simulink model "DiagnosPipeline"  (R2023b)
settings: Solver=VariableStepAuto  StartTime=0.0  StopTime=10.0  RelTol=1e-3
model workspace (MAT data in the model file):
  Signal = Simulink.ValueType
  Signal.Unit = 'V'
settings Model: Creator=user  LastModifiedBy=user

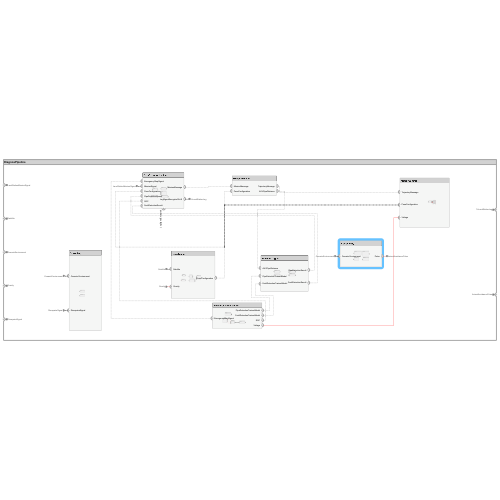
[thumbnail: Simulink's stored preview of the top-level diagram]
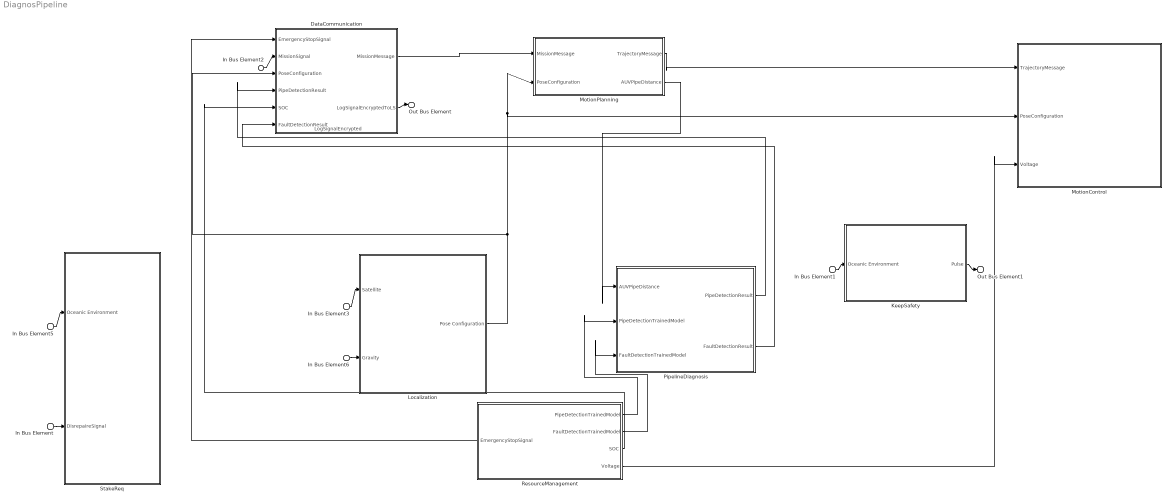
== system DiagnosPipeline ==
  In Bus Element2 : Inport  PortName=LandStationMissionSignal
  In Bus Element3 : Inport  Port=2  PortName=Satellite
  In Bus Element1 : Inport  Port=3  PortName=OceanicEnvironment
  In Bus Element5 : Inport  Port=3  PortName=OceanicEnvironment
  In Bus Element6 : Inport  Port=4  PortName=Gravity
  In Bus Element : Inport  Port=5  PortName=DisrepaireSignal
  DataCommunication : Subsystem
      settings: PortSchema="{\"entries\":[{\"content\":{\"headerSize\":26,\"margin\":15,\"minimumSpacing\":25,\"sides\":[{\"content\":{\"connectorIds\":[\"In7\",\"In2\",\"In3\",\"In4\",\"In5\",\"In6\"]},\"type\":\"ConnectorPlacement.EquallySpacedRectSide\",\"uuid\":\"b3d58345-43be-4317-860a-c8f4bed21ded\"},{\"content\":{\"connectorIds\":[\"Out1\",\"Out2\"],\"side\":\"RIGHT\"},\"type\":\"ConnectorPlacement.EquallySpacedRectSide\",\"uuid\":\"08e8d4ff-ef02-4699-9445-63f561e5af0c\"},{\"content\":{\"side\":\"TOP\"},\"type\":\"ConnectorPlacement.EquallySpacedRectSide\",\"uuid\":\"7d1ef7df-3e88-4641-86fc-bf7d4b5fe69f\"},{\"content\":{\"connectorIds\":[\"In1\"],\"side\":\"BOTTOM\"},\"type\":\"ConnectorPlacement.EquallySpacedRectSide\",\"uuid\":\"bd1e44a0-91aa-4375-ad49-10f8b22e6d3f\"}]},\"type\":\"ConnectorPlacement.EquallySpacedConnector\",\"uuid\":\"d738e7d3-0b43-4bd6-b335-43d88195508e\"}],\"packageUris\":[\"http://schema.mathworks.com/mf0/Connector/R2020b\"],\"version\":\"1.0\"}"
  KeepSafety : Subsystem
      settings: PortSchema="{\"entries\":[{\"content\":{\"headerSize\":26,\"margin\":15,\"minimumSpacing\":25,\"sides\":[{\"content\":{\"connectorIds\":[\"In1\"]},\"type\":\"ConnectorPlacement.EquallySpacedRectSide\",\"uuid\":\"b3d58345-43be-4317-860a-c8f4bed21ded\"},{\"content\":{\"connectorIds\":[\"Out1\"],\"side\":\"RIGHT\"},\"type\":\"ConnectorPlacement.EquallySpacedRectSide\",\"uuid\":\"08e8d4ff-ef02-4699-9445-63f561e5af0c\"},{\"content\":{\"side\":\"TOP\"},\"type\":\"ConnectorPlacement.EquallySpacedRectSide\",\"uuid\":\"7d1ef7df-3e88-4641-86fc-bf7d4b5fe69f\"}]},\"type\":\"ConnectorPlacement.EquallySpacedConnector\",\"uuid\":\"d738e7d3-0b43-4bd6-b335-43d88195508e\"}],\"packageUris\":[\"http://schema.mathworks.com/mf0/Connector/R2020b\"],\"version\":\"1.0\"}"
  Localization : Subsystem
      settings: PortSchema="{\"entries\":[{\"content\":{\"headerSize\":26,\"margin\":15,\"minimumSpacing\":25,\"sides\":[{\"content\":{\"connectorIds\":[\"In1\",\"In2\"]},\"type\":\"ConnectorPlacement.EquallySpacedRectSide\",\"uuid\":\"b3d58345-43be-4317-860a-c8f4bed21ded\"},{\"content\":{\"connectorIds\":[\"Out1\"],\"side\":\"RIGHT\"},\"type\":\"ConnectorPlacement.EquallySpacedRectSide\",\"uuid\":\"08e8d4ff-ef02-4699-9445-63f561e5af0c\"},{\"content\":{\"side\":\"TOP\"},\"type\":\"ConnectorPlacement.EquallySpacedRectSide\",\"uuid\":\"7d1ef7df-3e88-4641-86fc-bf7d4b5fe69f\"}]},\"type\":\"ConnectorPlacement.EquallySpacedConnector\",\"uuid\":\"d738e7d3-0b43-4bd6-b335-43d88195508e\"}],\"packageUris\":[\"http://schema.mathworks.com/mf0/Connector/R2020b\"],\"version\":\"1.0\"}"
  MotionControl : Subsystem
      settings: PortSchema="{\"entries\":[{\"content\":{\"headerSize\":26,\"margin\":15,\"minimumSpacing\":25,\"sides\":[{\"content\":{\"connectorIds\":[\"In1\",\"In2\",\"In3\"]},\"type\":\"ConnectorPlacement.EquallySpacedRectSide\",\"uuid\":\"2febbb42-d1b9-4a88-a98c-82119c43dfae\"},{\"content\":{\"side\":\"RIGHT\"},\"type\":\"ConnectorPlacement.EquallySpacedRectSide\",\"uuid\":\"6c566bdb-e273-46e8-952f-8993688d3046\"},{\"content\":{\"side\":\"TOP\"},\"type\":\"ConnectorPlacement.EquallySpacedRectSide\",\"uuid\":\"e45a7293-b6d9-4b29-b5bd-510d1f0460b1\"}]},\"type\":\"ConnectorPlacement.EquallySpacedConnector\",\"uuid\":\"1be34787-3cbc-414b-91e0-fdbde8ab0ed9\"}],\"packageUris\":[\"http://schema.mathworks.com/mf0/Connector/R2020b\"],\"version\":\"1.0\"}"
  MotionPlanning : Subsystem
      settings: PortSchema="{\"entries\":[{\"content\":{\"headerSize\":26,\"margin\":15,\"minimumSpacing\":25,\"sides\":[{\"content\":{\"connectorIds\":[\"In1\",\"In2\"]},\"type\":\"ConnectorPlacement.EquallySpacedRectSide\",\"uuid\":\"b3d58345-43be-4317-860a-c8f4bed21ded\"},{\"content\":{\"connectorIds\":[\"Out1\",\"Out2\"],\"side\":\"RIGHT\"},\"type\":\"ConnectorPlacement.EquallySpacedRectSide\",\"uuid\":\"08e8d4ff-ef02-4699-9445-63f561e5af0c\"},{\"content\":{\"side\":\"TOP\"},\"type\":\"ConnectorPlacement.EquallySpacedRectSide\",\"uuid\":\"7d1ef7df-3e88-4641-86fc-bf7d4b5fe69f\"}]},\"type\":\"ConnectorPlacement.EquallySpacedConnector\",\"uuid\":\"d738e7d3-0b43-4bd6-b335-43d88195508e\"}],\"packageUris\":[\"http://schema.mathworks.com/mf0/Connector/R2020b\"],\"version\":\"1.0\"}"
  PipelineDiagnosis : Subsystem
      settings: PortSchema="{\"entries\":[{\"content\":{\"headerSize\":26,\"margin\":15,\"minimumSpacing\":25,\"sides\":[{\"content\":{\"connectorIds\":[\"In1\",\"In2\",\"In3\"]},\"type\":\"ConnectorPlacement.EquallySpacedRectSide\",\"uuid\":\"b3d58345-43be-4317-860a-c8f4bed21ded\"},{\"content\":{\"connectorIds\":[\"Out1\",\"Out2\"],\"side\":\"RIGHT\"},\"type\":\"ConnectorPlacement.EquallySpacedRectSide\",\"uuid\":\"08e8d4ff-ef02-4699-9445-63f561e5af0c\"},{\"content\":{\"side\":\"TOP\"},\"type\":\"ConnectorPlacement.EquallySpacedRectSide\",\"uuid\":\"7d1ef7df-3e88-4641-86fc-bf7d4b5fe69f\"}]},\"type\":\"ConnectorPlacement.EquallySpacedConnector\",\"uuid\":\"d738e7d3-0b43-4bd6-b335-43d88195508e\"}],\"packageUris\":[\"http://schema.mathworks.com/mf0/Connector/R2020b\"],\"version\":\"1.0\"}"
  ResourceManagement : Subsystem
      settings: PortSchema="{\"entries\":[{\"content\":{\"headerSize\":26,\"margin\":15,\"minimumSpacing\":25,\"sides\":[{\"content\":{\"connectorIds\":[\"Out5\"]},\"type\":\"ConnectorPlacement.EquallySpacedRectSide\",\"uuid\":\"b3d58345-43be-4317-860a-c8f4bed21ded\"},{\"content\":{\"connectorIds\":[\"Out1\",\"Out2\",\"Out3\",\"Out4\"],\"side\":\"RIGHT\"},\"type\":\"ConnectorPlacement.EquallySpacedRectSide\",\"uuid\":\"08e8d4ff-ef02-4699-9445-63f561e5af0c\"},{\"content\":{\"side\":\"TOP\"},\"type\":\"ConnectorPlacement.EquallySpacedRectSide\",\"uuid\":\"7d1ef7df-3e88-4641-86fc-bf7d4b5fe69f\"}]},\"type\":\"ConnectorPlacement.EquallySpacedConnector\",\"uuid\":\"d738e7d3-0b43-4bd6-b335-43d88195508e\"}],\"packageUris\":[\"http://schema.mathworks.com/mf0/Connector/R2020b\"],\"version\":\"1.0\"}"
  StakeReq : Subsystem
      settings: PortSchema="{\"entries\":[{\"content\":{\"headerSize\":26,\"margin\":15,\"minimumSpacing\":25,\"sides\":[{\"content\":{\"connectorIds\":[\"In1\",\"In2\"]},\"type\":\"ConnectorPlacement.EquallySpacedRectSide\",\"uuid\":\"f9fadc38-a5ed-4d2c-8740-325682f7523a\"},{\"content\":{\"side\":\"RIGHT\"},\"type\":\"ConnectorPlacement.EquallySpacedRectSide\",\"uuid\":\"4cbd6435-b8f9-40e4-9703-696d88d9d9ae\"},{\"content\":{\"side\":\"TOP\"},\"type\":\"ConnectorPlacement.EquallySpacedRectSide\",\"uuid\":\"4cdd59a8-5a6d-4988-b682-29bfa74ce39c\"}]},\"type\":\"ConnectorPlacement.EquallySpacedConnector\",\"uuid\":\"f6db6523-916a-4ed8-a308-4b7cb9d0bc19\"}],\"packageUris\":[\"http://schema.mathworks.com/mf0/Connector/R2020b\"],\"version\":\"1.0\"}"
  Out Bus Element : Outport  PortName=ToLandStationLog
  Out Bus Element1 : Outport  Port=2  PortName=AnimalAvoidancePulse
  wires:
  Localization/1(Pose Configuration) -> MotionControl/2(PoseConfiguration), MotionPlanning/2(PoseConfiguration), DataCommunication/3(PoseConfiguration)
  In Bus Element2/1 -> DataCommunication/2(MissionSignal)
  In Bus Element3/1 -> Localization/1(Satellite)
  PipelineDiagnosis/1(PipeDetectionResult) -> DataCommunication/4(PipeDetectionResult)
  PipelineDiagnosis/2(FaultDetectionResult) -> DataCommunication/6(FaultDetectionResult)
  ResourceManagement/1(PipeDetectionTrainedModel) -> PipelineDiagnosis/2(PipeDetectionTrainedModel)
  ResourceManagement/2(FaultDetectionTrainedModel) -> PipelineDiagnosis/3(FaultDetectionTrainedModel)
  ResourceManagement/5(EmergencyStopSignal) -> DataCommunication/7(EmergencyStopSignal)
  KeepSafety/1(Pulse) -> Out Bus Element1/1
  DataCommunication/1(MissionMessage) -> MotionPlanning/1(MissionMessage)
  MotionPlanning/2(AUVPipeDistance) -> PipelineDiagnosis/1(AUVPipeDistance)
  MotionPlanning/1(TrajectoryMessage) -> MotionControl/1(TrajectoryMessage)
  ResourceManagement/4(Voltage) -> MotionControl/3(Voltage)
  In Bus Element1/1 -> KeepSafety/1(Oceanic Environment)
  In Bus Element5/1 -> StakeReq/1(Oceanic Environment)
  In Bus Element/1 -> StakeReq/2(DisrepaireSignal)
  DataCommunication/2(LogSignalEncryptedToLS) -> Out Bus Element/1
  In Bus Element6/1 -> Localization/2(Gravity)
  ResourceManagement/3(SOC) -> DataCommunication/5(SOC)

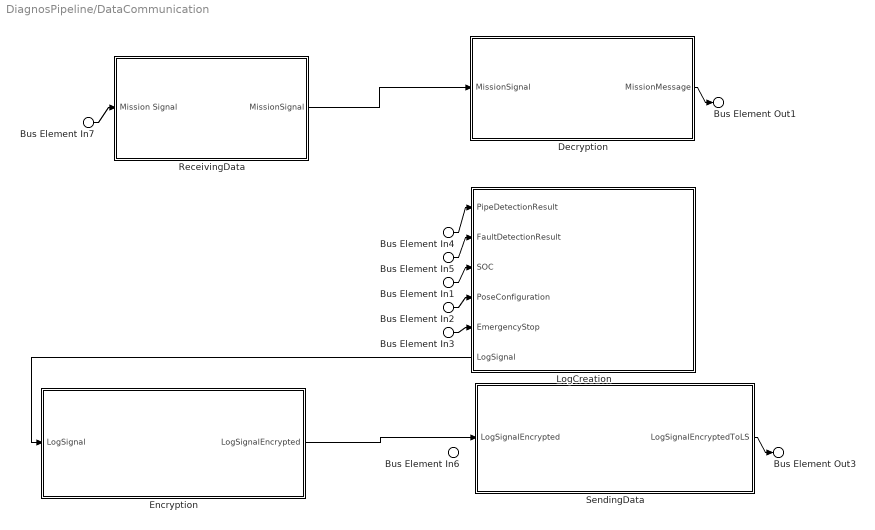
== system DiagnosPipeline/DataCommunication ==
  Bus Element In6 : Inport  PortName=LogSignalEncrypted
  Bus Element In7 : Inport  Port=2  PortName=MissionSignal
  Bus Element In2 : Inport  Port=3  PortName=PoseConfiguration
  Bus Element In4 : Inport  Port=4  PortName=PipeDetectionResult
  Bus Element In1 : Inport  Port=5  PortName=SOC
  Bus Element In5 : Inport  Port=6  PortName=FaultDetectionResult
  Bus Element In3 : Inport  Port=7  PortName=EmergencyStopSignal
  Decryption : Subsystem
      settings: PortSchema="{\"entries\":[{\"content\":{\"headerSize\":26,\"margin\":15,\"minimumSpacing\":25,\"sides\":[{\"content\":{\"connectorIds\":[\"In1\"]},\"type\":\"ConnectorPlacement.EquallySpacedRectSide\",\"uuid\":\"e6d1833a-8836-49de-81ae-600a650351e4\"},{\"content\":{\"connectorIds\":[\"Out1\"],\"side\":\"RIGHT\"},\"type\":\"ConnectorPlacement.EquallySpacedRectSide\",\"uuid\":\"f245f6bb-811b-4e93-b151-5c323e86052c\"},{\"content\":{\"side\":\"TOP\"},\"type\":\"ConnectorPlacement.EquallySpacedRectSide\",\"uuid\":\"48a167ed-d4c2-4e7f-a44b-e328bb65996f\"}]},\"type\":\"ConnectorPlacement.EquallySpacedConnector\",\"uuid\":\"b7272ec2-108a-4004-85a9-2681fa300cc3\"}],\"packageUris\":[\"http://schema.mathworks.com/mf0/Connector/R2020b\"],\"version\":\"1.0\"}"
  Encryption : Subsystem
      settings: PortSchema="{\"entries\":[{\"content\":{\"headerSize\":26,\"margin\":15,\"minimumSpacing\":25,\"sides\":[{\"content\":{\"connectorIds\":[\"In1\"]},\"type\":\"ConnectorPlacement.EquallySpacedRectSide\",\"uuid\":\"e6d1833a-8836-49de-81ae-600a650351e4\"},{\"content\":{\"connectorIds\":[\"Out1\"],\"side\":\"RIGHT\"},\"type\":\"ConnectorPlacement.EquallySpacedRectSide\",\"uuid\":\"f245f6bb-811b-4e93-b151-5c323e86052c\"},{\"content\":{\"side\":\"TOP\"},\"type\":\"ConnectorPlacement.EquallySpacedRectSide\",\"uuid\":\"48a167ed-d4c2-4e7f-a44b-e328bb65996f\"}]},\"type\":\"ConnectorPlacement.EquallySpacedConnector\",\"uuid\":\"b7272ec2-108a-4004-85a9-2681fa300cc3\"}],\"packageUris\":[\"http://schema.mathworks.com/mf0/Connector/R2020b\"],\"version\":\"1.0\"}"
  LogCreation : Subsystem
      settings: PortSchema="{\"entries\":[{\"content\":{\"headerSize\":26,\"margin\":15,\"minimumSpacing\":25,\"sides\":[{\"content\":{\"connectorIds\":[\"In1\",\"In2\",\"In3\",\"In4\",\"In5\",\"Out1\"]},\"type\":\"ConnectorPlacement.EquallySpacedRectSide\",\"uuid\":\"e6d1833a-8836-49de-81ae-600a650351e4\"},{\"content\":{\"side\":\"RIGHT\"},\"type\":\"ConnectorPlacement.EquallySpacedRectSide\",\"uuid\":\"f245f6bb-811b-4e93-b151-5c323e86052c\"},{\"content\":{\"side\":\"TOP\"},\"type\":\"ConnectorPlacement.EquallySpacedRectSide\",\"uuid\":\"48a167ed-d4c2-4e7f-a44b-e328bb65996f\"}]},\"type\":\"ConnectorPlacement.EquallySpacedConnector\",\"uuid\":\"b7272ec2-108a-4004-85a9-2681fa300cc3\"}],\"packageUris\":[\"http://schema.mathworks.com/mf0/Connector/R2020b\"],\"version\":\"1.0\"}"
  ReceivingData : Subsystem
      settings: PortSchema="{\"entries\":[{\"content\":{\"headerSize\":26,\"margin\":15,\"minimumSpacing\":25,\"sides\":[{\"content\":{\"connectorIds\":[\"In1\"]},\"type\":\"ConnectorPlacement.EquallySpacedRectSide\",\"uuid\":\"f9fadc38-a5ed-4d2c-8740-325682f7523a\"},{\"content\":{\"connectorIds\":[\"Out1\"],\"side\":\"RIGHT\"},\"type\":\"ConnectorPlacement.EquallySpacedRectSide\",\"uuid\":\"4cbd6435-b8f9-40e4-9703-696d88d9d9ae\"},{\"content\":{\"side\":\"TOP\"},\"type\":\"ConnectorPlacement.EquallySpacedRectSide\",\"uuid\":\"4cdd59a8-5a6d-4988-b682-29bfa74ce39c\"}]},\"type\":\"ConnectorPlacement.EquallySpacedConnector\",\"uuid\":\"f6db6523-916a-4ed8-a308-4b7cb9d0bc19\"}],\"packageUris\":[\"http://schema.mathworks.com/mf0/Connector/R2020b\"],\"version\":\"1.0\"}"
  SendingData : Subsystem
      settings: PortSchema="{\"entries\":[{\"content\":{\"headerSize\":26,\"margin\":15,\"minimumSpacing\":25,\"sides\":[{\"content\":{\"connectorIds\":[\"In1\"]},\"type\":\"ConnectorPlacement.EquallySpacedRectSide\",\"uuid\":\"f9fadc38-a5ed-4d2c-8740-325682f7523a\"},{\"content\":{\"connectorIds\":[\"Out1\"],\"side\":\"RIGHT\"},\"type\":\"ConnectorPlacement.EquallySpacedRectSide\",\"uuid\":\"4cbd6435-b8f9-40e4-9703-696d88d9d9ae\"},{\"content\":{\"side\":\"TOP\"},\"type\":\"ConnectorPlacement.EquallySpacedRectSide\",\"uuid\":\"4cdd59a8-5a6d-4988-b682-29bfa74ce39c\"}]},\"type\":\"ConnectorPlacement.EquallySpacedConnector\",\"uuid\":\"f6db6523-916a-4ed8-a308-4b7cb9d0bc19\"}],\"packageUris\":[\"http://schema.mathworks.com/mf0/Connector/R2020b\"],\"version\":\"1.0\"}"
  Bus Element Out1 : Outport  PortName=MissionMessage
  Bus Element Out3 : Outport  Port=2  PortName=LogSignalEncryptedToLS
  wires:
  Decryption/1(MissionMessage) -> Bus Element Out1/1
  Bus Element In2/1 -> LogCreation/4(PoseConfiguration)
  Bus Element In4/1 -> LogCreation/1(PipeDetectionResult)
  Bus Element In5/1 -> LogCreation/2(FaultDetectionResult)
  Bus Element In3/1 -> LogCreation/5(EmergencyStop)
  Bus Element In7/1 -> ReceivingData/1(Mission Signal)
  ReceivingData/1(MissionSignal) -> Decryption/1(MissionSignal)
  SendingData/1(LogSignalEncryptedToLS) -> Bus Element Out3/1
  LogCreation/1(LogSignal) -> Encryption/1(LogSignal)
  Encryption/1(LogSignalEncrypted) -> SendingData/1(LogSignalEncrypted)
  Bus Element In1/1 -> LogCreation/3(SOC)

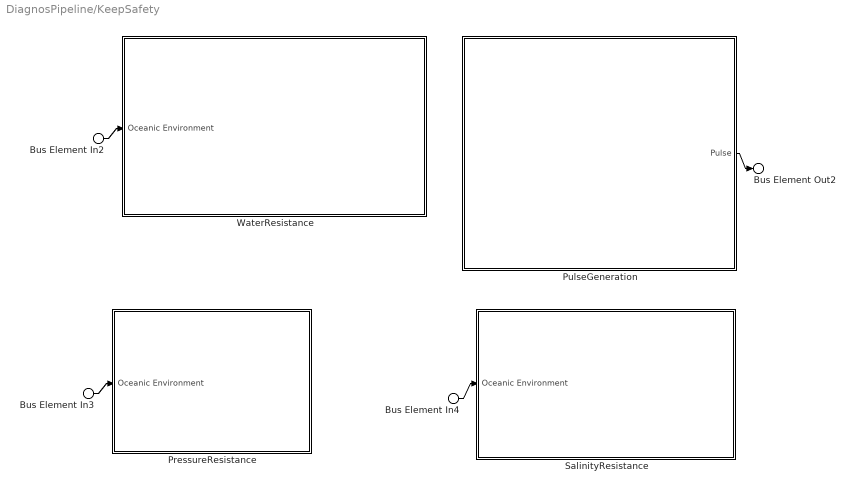
== system DiagnosPipeline/KeepSafety ==
  Bus Element In2 : Inport  PortName=Oceanic Environment
  Bus Element In3 : Inport  PortName=Oceanic Environment
  Bus Element In4 : Inport  PortName=Oceanic Environment
  PressureResistance : Subsystem
      settings: PortSchema="{\"entries\":[{\"content\":{\"headerSize\":26,\"margin\":15,\"minimumSpacing\":25,\"sides\":[{\"content\":{\"connectorIds\":[\"In1\"]},\"type\":\"ConnectorPlacement.EquallySpacedRectSide\",\"uuid\":\"f9fadc38-a5ed-4d2c-8740-325682f7523a\"},{\"content\":{\"side\":\"RIGHT\"},\"type\":\"ConnectorPlacement.EquallySpacedRectSide\",\"uuid\":\"4cbd6435-b8f9-40e4-9703-696d88d9d9ae\"},{\"content\":{\"side\":\"TOP\"},\"type\":\"ConnectorPlacement.EquallySpacedRectSide\",\"uuid\":\"4cdd59a8-5a6d-4988-b682-29bfa74ce39c\"}]},\"type\":\"ConnectorPlacement.EquallySpacedConnector\",\"uuid\":\"f6db6523-916a-4ed8-a308-4b7cb9d0bc19\"}],\"packageUris\":[\"http://schema.mathworks.com/mf0/Connector/R2020b\"],\"version\":\"1.0\"}"
  PulseGeneration : Subsystem
      settings: PortSchema="{\"entries\":[{\"content\":{\"headerSize\":26,\"margin\":15,\"minimumSpacing\":25,\"sides\":[{\"content\":{},\"type\":\"ConnectorPlacement.EquallySpacedRectSide\",\"uuid\":\"e6d1833a-8836-49de-81ae-600a650351e4\"},{\"content\":{\"connectorIds\":[\"Out1\"],\"side\":\"RIGHT\"},\"type\":\"ConnectorPlacement.EquallySpacedRectSide\",\"uuid\":\"f245f6bb-811b-4e93-b151-5c323e86052c\"},{\"content\":{\"side\":\"TOP\"},\"type\":\"ConnectorPlacement.EquallySpacedRectSide\",\"uuid\":\"48a167ed-d4c2-4e7f-a44b-e328bb65996f\"}]},\"type\":\"ConnectorPlacement.EquallySpacedConnector\",\"uuid\":\"b7272ec2-108a-4004-85a9-2681fa300cc3\"}],\"packageUris\":[\"http://schema.mathworks.com/mf0/Connector/R2020b\"],\"version\":\"1.0\"}"
  SalinityResistance : Subsystem
      settings: PortSchema="{\"entries\":[{\"content\":{\"headerSize\":26,\"margin\":15,\"minimumSpacing\":25,\"sides\":[{\"content\":{\"connectorIds\":[\"In1\"]},\"type\":\"ConnectorPlacement.EquallySpacedRectSide\",\"uuid\":\"f9fadc38-a5ed-4d2c-8740-325682f7523a\"},{\"content\":{\"side\":\"RIGHT\"},\"type\":\"ConnectorPlacement.EquallySpacedRectSide\",\"uuid\":\"4cbd6435-b8f9-40e4-9703-696d88d9d9ae\"},{\"content\":{\"side\":\"TOP\"},\"type\":\"ConnectorPlacement.EquallySpacedRectSide\",\"uuid\":\"4cdd59a8-5a6d-4988-b682-29bfa74ce39c\"}]},\"type\":\"ConnectorPlacement.EquallySpacedConnector\",\"uuid\":\"f6db6523-916a-4ed8-a308-4b7cb9d0bc19\"}],\"packageUris\":[\"http://schema.mathworks.com/mf0/Connector/R2020b\"],\"version\":\"1.0\"}"
  WaterResistance : Subsystem
      settings: PortSchema="{\"entries\":[{\"content\":{\"headerSize\":26,\"margin\":15,\"minimumSpacing\":25,\"sides\":[{\"content\":{\"connectorIds\":[\"In1\"]},\"type\":\"ConnectorPlacement.EquallySpacedRectSide\",\"uuid\":\"f9fadc38-a5ed-4d2c-8740-325682f7523a\"},{\"content\":{\"side\":\"RIGHT\"},\"type\":\"ConnectorPlacement.EquallySpacedRectSide\",\"uuid\":\"4cbd6435-b8f9-40e4-9703-696d88d9d9ae\"},{\"content\":{\"side\":\"TOP\"},\"type\":\"ConnectorPlacement.EquallySpacedRectSide\",\"uuid\":\"4cdd59a8-5a6d-4988-b682-29bfa74ce39c\"}]},\"type\":\"ConnectorPlacement.EquallySpacedConnector\",\"uuid\":\"f6db6523-916a-4ed8-a308-4b7cb9d0bc19\"}],\"packageUris\":[\"http://schema.mathworks.com/mf0/Connector/R2020b\"],\"version\":\"1.0\"}"
  Bus Element Out2 : Outport  PortName=Pulse
  wires:
  PulseGeneration/1(Pulse) -> Bus Element Out2/1
  Bus Element In2/1 -> WaterResistance/1(Oceanic Environment)
  Bus Element In3/1 -> PressureResistance/1(Oceanic Environment)
  Bus Element In4/1 -> SalinityResistance/1(Oceanic Environment)

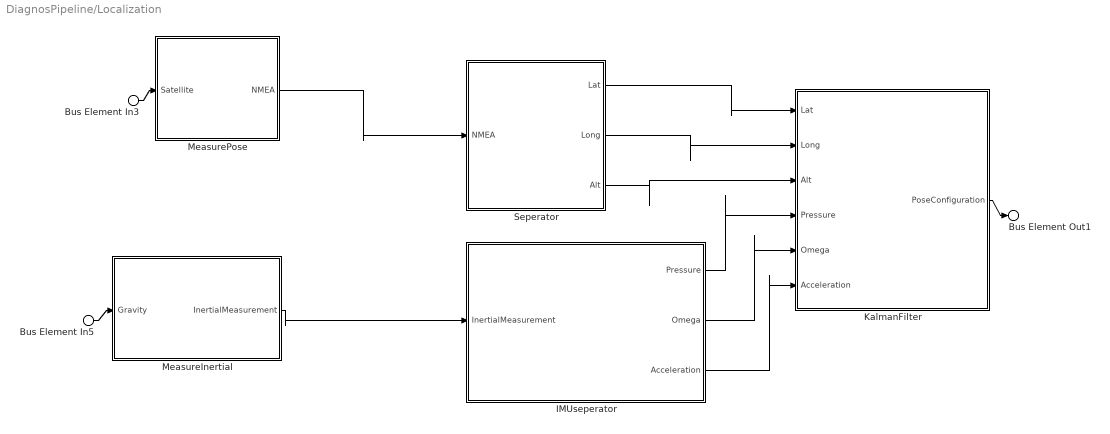
== system DiagnosPipeline/Localization ==
  Bus Element In3 : Inport  PortName=Satellite
  Bus Element In5 : Inport  Port=2  PortName=Gravity
  IMUseperator : Subsystem
      settings: PortSchema="{\"entries\":[{\"content\":{\"headerSize\":26,\"margin\":15,\"minimumSpacing\":25,\"sides\":[{\"content\":{\"connectorIds\":[\"In1\"]},\"type\":\"ConnectorPlacement.EquallySpacedRectSide\",\"uuid\":\"e6d1833a-8836-49de-81ae-600a650351e4\"},{\"content\":{\"connectorIds\":[\"Out1\",\"Out2\",\"Out3\"],\"side\":\"RIGHT\"},\"type\":\"ConnectorPlacement.EquallySpacedRectSide\",\"uuid\":\"f245f6bb-811b-4e93-b151-5c323e86052c\"},{\"content\":{\"side\":\"TOP\"},\"type\":\"ConnectorPlacement.EquallySpacedRectSide\",\"uuid\":\"48a167ed-d4c2-4e7f-a44b-e328bb65996f\"}]},\"type\":\"ConnectorPlacement.EquallySpacedConnector\",\"uuid\":\"b7272ec2-108a-4004-85a9-2681fa300cc3\"}],\"packageUris\":[\"http://schema.mathworks.com/mf0/Connector/R2020b\"],\"version\":\"1.0\"}"
  KalmanFilter : Subsystem
      settings: PortSchema="{\"entries\":[{\"content\":{\"headerSize\":26,\"margin\":15,\"minimumSpacing\":25,\"sides\":[{\"content\":{\"connectorIds\":[\"In1\",\"In2\",\"In3\",\"In4\",\"In5\",\"In6\"]},\"type\":\"ConnectorPlacement.EquallySpacedRectSide\",\"uuid\":\"e6d1833a-8836-49de-81ae-600a650351e4\"},{\"content\":{\"connectorIds\":[\"Out1\"],\"side\":\"RIGHT\"},\"type\":\"ConnectorPlacement.EquallySpacedRectSide\",\"uuid\":\"f245f6bb-811b-4e93-b151-5c323e86052c\"},{\"content\":{\"side\":\"TOP\"},\"type\":\"ConnectorPlacement.EquallySpacedRectSide\",\"uuid\":\"48a167ed-d4c2-4e7f-a44b-e328bb65996f\"}]},\"type\":\"ConnectorPlacement.EquallySpacedConnector\",\"uuid\":\"b7272ec2-108a-4004-85a9-2681fa300cc3\"}],\"packageUris\":[\"http://schema.mathworks.com/mf0/Connector/R2020b\"],\"version\":\"1.0\"}"
  MeasureInertial : Subsystem
      settings: PortSchema="{\"entries\":[{\"content\":{\"headerSize\":26,\"margin\":15,\"minimumSpacing\":25,\"sides\":[{\"content\":{\"connectorIds\":[\"In1\"]},\"type\":\"ConnectorPlacement.EquallySpacedRectSide\",\"uuid\":\"f9fadc38-a5ed-4d2c-8740-325682f7523a\"},{\"content\":{\"connectorIds\":[\"Out1\"],\"side\":\"RIGHT\"},\"type\":\"ConnectorPlacement.EquallySpacedRectSide\",\"uuid\":\"4cbd6435-b8f9-40e4-9703-696d88d9d9ae\"},{\"content\":{\"side\":\"TOP\"},\"type\":\"ConnectorPlacement.EquallySpacedRectSide\",\"uuid\":\"4cdd59a8-5a6d-4988-b682-29bfa74ce39c\"}]},\"type\":\"ConnectorPlacement.EquallySpacedConnector\",\"uuid\":\"f6db6523-916a-4ed8-a308-4b7cb9d0bc19\"}],\"packageUris\":[\"http://schema.mathworks.com/mf0/Connector/R2020b\"],\"version\":\"1.0\"}"
  MeasurePose : Subsystem
      settings: PortSchema="{\"entries\":[{\"content\":{\"headerSize\":26,\"margin\":15,\"minimumSpacing\":25,\"sides\":[{\"content\":{\"connectorIds\":[\"In1\"]},\"type\":\"ConnectorPlacement.EquallySpacedRectSide\",\"uuid\":\"f9fadc38-a5ed-4d2c-8740-325682f7523a\"},{\"content\":{\"connectorIds\":[\"Out1\"],\"side\":\"RIGHT\"},\"type\":\"ConnectorPlacement.EquallySpacedRectSide\",\"uuid\":\"4cbd6435-b8f9-40e4-9703-696d88d9d9ae\"},{\"content\":{\"side\":\"TOP\"},\"type\":\"ConnectorPlacement.EquallySpacedRectSide\",\"uuid\":\"4cdd59a8-5a6d-4988-b682-29bfa74ce39c\"}]},\"type\":\"ConnectorPlacement.EquallySpacedConnector\",\"uuid\":\"f6db6523-916a-4ed8-a308-4b7cb9d0bc19\"}],\"packageUris\":[\"http://schema.mathworks.com/mf0/Connector/R2020b\"],\"version\":\"1.0\"}"
  Seperator : Subsystem
      settings: PortSchema="{\"entries\":[{\"content\":{\"headerSize\":26,\"margin\":15,\"minimumSpacing\":25,\"sides\":[{\"content\":{\"connectorIds\":[\"In1\"]},\"type\":\"ConnectorPlacement.EquallySpacedRectSide\",\"uuid\":\"e6d1833a-8836-49de-81ae-600a650351e4\"},{\"content\":{\"connectorIds\":[\"Out1\",\"Out2\",\"Out3\"],\"side\":\"RIGHT\"},\"type\":\"ConnectorPlacement.EquallySpacedRectSide\",\"uuid\":\"f245f6bb-811b-4e93-b151-5c323e86052c\"},{\"content\":{\"side\":\"TOP\"},\"type\":\"ConnectorPlacement.EquallySpacedRectSide\",\"uuid\":\"48a167ed-d4c2-4e7f-a44b-e328bb65996f\"}]},\"type\":\"ConnectorPlacement.EquallySpacedConnector\",\"uuid\":\"b7272ec2-108a-4004-85a9-2681fa300cc3\"}],\"packageUris\":[\"http://schema.mathworks.com/mf0/Connector/R2020b\"],\"version\":\"1.0\"}"
  Bus Element Out1 : Outport  PortName=Pose Configuration
  wires:
  KalmanFilter/1(PoseConfiguration) -> Bus Element Out1/1
  Seperator/1(Lat) -> KalmanFilter/1(Lat)
  Seperator/2(Long) -> KalmanFilter/2(Long)
  Seperator/3(Alt) -> KalmanFilter/3(Alt)
  IMUseperator/1(Pressure) -> KalmanFilter/4(Pressure)
  IMUseperator/2(Omega) -> KalmanFilter/5(Omega)
  IMUseperator/3(Acceleration) -> KalmanFilter/6(Acceleration)
  Bus Element In3/1 -> MeasurePose/1(Satellite)
  Bus Element In5/1 -> MeasureInertial/1(Gravity)
  MeasurePose/1(NMEA) -> Seperator/1(NMEA)
  MeasureInertial/1(InertialMeasurement) -> IMUseperator/1(InertialMeasurement)

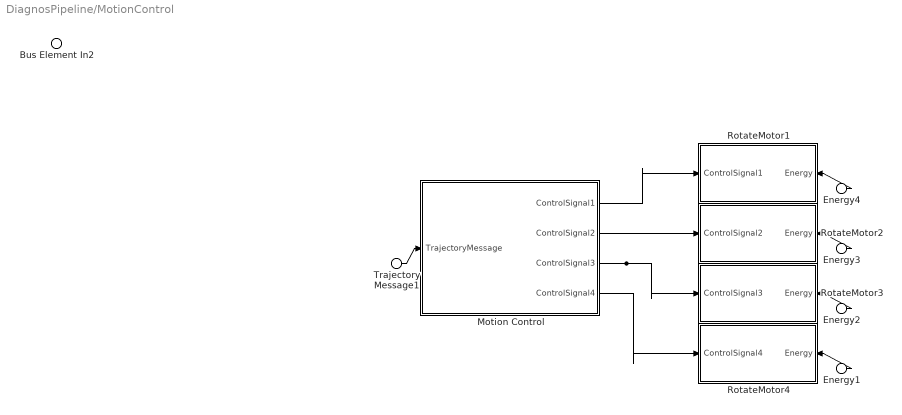
== system DiagnosPipeline/MotionControl ==
  Trajectory Message1 : Inport  PortName=TrajectoryMessage
  Bus Element In2 : Inport  Port=2  PortName=PoseConfiguration
  Energy{1..4} (4 alike) : Inport  Port=3  PortName=Voltage
  Motion Control : Subsystem
      settings: PortSchema="{\"entries\":[{\"content\":{\"headerSize\":26,\"margin\":15,\"minimumSpacing\":25,\"sides\":[{\"content\":{\"connectorIds\":[\"In1\"]},\"type\":\"ConnectorPlacement.EquallySpacedRectSide\",\"uuid\":\"b3d58345-43be-4317-860a-c8f4bed21ded\"},{\"content\":{\"connectorIds\":[\"Out1\",\"Out2\",\"Out3\",\"Out4\"],\"side\":\"RIGHT\"},\"type\":\"ConnectorPlacement.EquallySpacedRectSide\",\"uuid\":\"08e8d4ff-ef02-4699-9445-63f561e5af0c\"},{\"content\":{\"side\":\"TOP\"},\"type\":\"ConnectorPlacement.EquallySpacedRectSide\",\"uuid\":\"7d1ef7df-3e88-4641-86fc-bf7d4b5fe69f\"}]},\"type\":\"ConnectorPlacement.EquallySpacedConnector\",\"uuid\":\"d738e7d3-0b43-4bd6-b335-43d88195508e\"}],\"packageUris\":[\"http://schema.mathworks.com/mf0/Connector/R2020b\"],\"version\":\"1.0\"}"
  RotateMotor1 : Subsystem
      settings: PortSchema="{\"entries\":[{\"content\":{\"headerSize\":26,\"margin\":15,\"minimumSpacing\":25,\"sides\":[{\"content\":{\"connectorIds\":[\"In2\"]},\"type\":\"ConnectorPlacement.EquallySpacedRectSide\",\"uuid\":\"b3d58345-43be-4317-860a-c8f4bed21ded\"},{\"content\":{\"connectorIds\":[\"In1\"],\"side\":\"RIGHT\"},\"type\":\"ConnectorPlacement.EquallySpacedRectSide\",\"uuid\":\"08e8d4ff-ef02-4699-9445-63f561e5af0c\"},{\"content\":{\"side\":\"TOP\"},\"type\":\"ConnectorPlacement.EquallySpacedRectSide\",\"uuid\":\"7d1ef7df-3e88-4641-86fc-bf7d4b5fe69f\"}]},\"type\":\"ConnectorPlacement.EquallySpacedConnector\",\"uuid\":\"d738e7d3-0b43-4bd6-b335-43d88195508e\"}],\"packageUris\":[\"http://schema.mathworks.com/mf0/Connector/R2020b\"],\"version\":\"1.0\"}"
  RotateMotor2 : Subsystem
      settings: PortSchema="{\"entries\":[{\"content\":{\"headerSize\":26,\"margin\":15,\"minimumSpacing\":25,\"sides\":[{\"content\":{\"connectorIds\":[\"In2\"]},\"type\":\"ConnectorPlacement.EquallySpacedRectSide\",\"uuid\":\"b3d58345-43be-4317-860a-c8f4bed21ded\"},{\"content\":{\"connectorIds\":[\"In1\"],\"side\":\"RIGHT\"},\"type\":\"ConnectorPlacement.EquallySpacedRectSide\",\"uuid\":\"08e8d4ff-ef02-4699-9445-63f561e5af0c\"},{\"content\":{\"side\":\"TOP\"},\"type\":\"ConnectorPlacement.EquallySpacedRectSide\",\"uuid\":\"7d1ef7df-3e88-4641-86fc-bf7d4b5fe69f\"}]},\"type\":\"ConnectorPlacement.EquallySpacedConnector\",\"uuid\":\"d738e7d3-0b43-4bd6-b335-43d88195508e\"}],\"packageUris\":[\"http://schema.mathworks.com/mf0/Connector/R2020b\"],\"version\":\"1.0\"}"
  RotateMotor3 : Subsystem
      settings: PortSchema="{\"entries\":[{\"content\":{\"headerSize\":26,\"margin\":15,\"minimumSpacing\":25,\"sides\":[{\"content\":{\"connectorIds\":[\"In2\"]},\"type\":\"ConnectorPlacement.EquallySpacedRectSide\",\"uuid\":\"b3d58345-43be-4317-860a-c8f4bed21ded\"},{\"content\":{\"connectorIds\":[\"In1\"],\"side\":\"RIGHT\"},\"type\":\"ConnectorPlacement.EquallySpacedRectSide\",\"uuid\":\"08e8d4ff-ef02-4699-9445-63f561e5af0c\"},{\"content\":{\"side\":\"TOP\"},\"type\":\"ConnectorPlacement.EquallySpacedRectSide\",\"uuid\":\"7d1ef7df-3e88-4641-86fc-bf7d4b5fe69f\"}]},\"type\":\"ConnectorPlacement.EquallySpacedConnector\",\"uuid\":\"d738e7d3-0b43-4bd6-b335-43d88195508e\"}],\"packageUris\":[\"http://schema.mathworks.com/mf0/Connector/R2020b\"],\"version\":\"1.0\"}"
  RotateMotor4 : Subsystem
      settings: PortSchema="{\"entries\":[{\"content\":{\"headerSize\":26,\"margin\":15,\"minimumSpacing\":25,\"sides\":[{\"content\":{\"connectorIds\":[\"In2\"]},\"type\":\"ConnectorPlacement.EquallySpacedRectSide\",\"uuid\":\"b3d58345-43be-4317-860a-c8f4bed21ded\"},{\"content\":{\"connectorIds\":[\"In1\"],\"side\":\"RIGHT\"},\"type\":\"ConnectorPlacement.EquallySpacedRectSide\",\"uuid\":\"08e8d4ff-ef02-4699-9445-63f561e5af0c\"},{\"content\":{\"side\":\"TOP\"},\"type\":\"ConnectorPlacement.EquallySpacedRectSide\",\"uuid\":\"7d1ef7df-3e88-4641-86fc-bf7d4b5fe69f\"}]},\"type\":\"ConnectorPlacement.EquallySpacedConnector\",\"uuid\":\"d738e7d3-0b43-4bd6-b335-43d88195508e\"}],\"packageUris\":[\"http://schema.mathworks.com/mf0/Connector/R2020b\"],\"version\":\"1.0\"}"
  wires:
  Motion Control/4(ControlSignal4) -> RotateMotor4/2(ControlSignal4)
  Motion Control/1(ControlSignal1) -> RotateMotor1/2(ControlSignal1)
  Motion Control/3(ControlSignal3) -> RotateMotor3/2(ControlSignal3)
  Motion Control/2(ControlSignal2) -> RotateMotor2/2(ControlSignal2)
  Energy1/1 -> RotateMotor4/1(Energy)
  Energy2/1 -> RotateMotor3/1(Energy)
  Energy3/1 -> RotateMotor2/1(Energy)
  Energy4/1 -> RotateMotor1/1(Energy)
  Trajectory Message1/1 -> Motion Control/1(TrajectoryMessage)

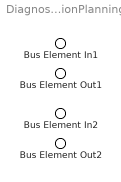
== system DiagnosPipeline/MotionPlanning ==
  Bus Element In1 : Inport  PortName=MissionMessage
  Bus Element In2 : Inport  Port=2  PortName=PoseConfiguration
  Bus Element Out1 : Outport  PortName=TrajectoryMessage
  Bus Element Out2 : Outport  Port=2  PortName=AUVPipeDistance

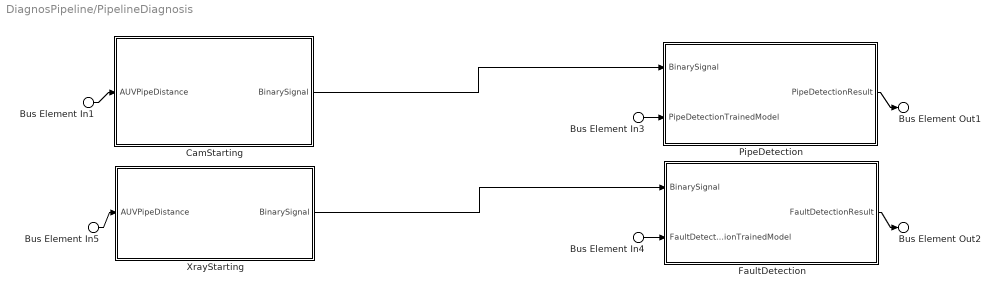
== system DiagnosPipeline/PipelineDiagnosis ==
  Bus Element In1 : Inport  PortName=AUVPipeDistance
  Bus Element In5 : Inport  PortName=AUVPipeDistance
  Bus Element In3 : Inport  Port=2  PortName=PipeDetectionTrainedModel
  Bus Element In4 : Inport  Port=3  PortName=FaultDetectionTrainedModel
  CamStarting : Subsystem
      settings: PortSchema="{\"entries\":[{\"content\":{\"headerSize\":26,\"margin\":15,\"minimumSpacing\":25,\"sides\":[{\"content\":{\"connectorIds\":[\"In1\"]},\"type\":\"ConnectorPlacement.EquallySpacedRectSide\",\"uuid\":\"e6d1833a-8836-49de-81ae-600a650351e4\"},{\"content\":{\"connectorIds\":[\"Out1\"],\"side\":\"RIGHT\"},\"type\":\"ConnectorPlacement.EquallySpacedRectSide\",\"uuid\":\"f245f6bb-811b-4e93-b151-5c323e86052c\"},{\"content\":{\"side\":\"TOP\"},\"type\":\"ConnectorPlacement.EquallySpacedRectSide\",\"uuid\":\"48a167ed-d4c2-4e7f-a44b-e328bb65996f\"}]},\"type\":\"ConnectorPlacement.EquallySpacedConnector\",\"uuid\":\"b7272ec2-108a-4004-85a9-2681fa300cc3\"}],\"packageUris\":[\"http://schema.mathworks.com/mf0/Connector/R2020b\"],\"version\":\"1.0\"}"
  FaultDetection : Subsystem
      settings: PortSchema="{\"entries\":[{\"content\":{\"headerSize\":26,\"margin\":15,\"minimumSpacing\":25,\"sides\":[{\"content\":{\"connectorIds\":[\"In1\",\"In2\"]},\"type\":\"ConnectorPlacement.EquallySpacedRectSide\",\"uuid\":\"e6d1833a-8836-49de-81ae-600a650351e4\"},{\"content\":{\"connectorIds\":[\"Out1\"],\"side\":\"RIGHT\"},\"type\":\"ConnectorPlacement.EquallySpacedRectSide\",\"uuid\":\"f245f6bb-811b-4e93-b151-5c323e86052c\"},{\"content\":{\"side\":\"TOP\"},\"type\":\"ConnectorPlacement.EquallySpacedRectSide\",\"uuid\":\"48a167ed-d4c2-4e7f-a44b-e328bb65996f\"}]},\"type\":\"ConnectorPlacement.EquallySpacedConnector\",\"uuid\":\"b7272ec2-108a-4004-85a9-2681fa300cc3\"}],\"packageUris\":[\"http://schema.mathworks.com/mf0/Connector/R2020b\"],\"version\":\"1.0\"}"
  PipeDetection : Subsystem
      settings: PortSchema="{\"entries\":[{\"content\":{\"headerSize\":26,\"margin\":15,\"minimumSpacing\":25,\"sides\":[{\"content\":{\"connectorIds\":[\"In1\",\"In2\"]},\"type\":\"ConnectorPlacement.EquallySpacedRectSide\",\"uuid\":\"e6d1833a-8836-49de-81ae-600a650351e4\"},{\"content\":{\"connectorIds\":[\"Out1\"],\"side\":\"RIGHT\"},\"type\":\"ConnectorPlacement.EquallySpacedRectSide\",\"uuid\":\"f245f6bb-811b-4e93-b151-5c323e86052c\"},{\"content\":{\"side\":\"TOP\"},\"type\":\"ConnectorPlacement.EquallySpacedRectSide\",\"uuid\":\"48a167ed-d4c2-4e7f-a44b-e328bb65996f\"},{\"content\":{\"side\":\"BOTTOM\"},\"type\":\"ConnectorPlacement.EquallySpacedRectSide\",\"uuid\":\"0104f4be-da01-4aa7-b92e-f862479c9d43\"}]},\"type\":\"ConnectorPlacement.EquallySpacedConnector\",\"uuid\":\"b7272ec2-108a-4004-85a9-2681fa300cc3\"}],\"packageUris\":[\"http://schema.mathworks.com/mf0/Connector/R2020b\"],\"version\":\"1.0\"}"
  XrayStarting : Subsystem
      settings: PortSchema="{\"entries\":[{\"content\":{\"headerSize\":26,\"margin\":15,\"minimumSpacing\":25,\"sides\":[{\"content\":{\"connectorIds\":[\"In1\"]},\"type\":\"ConnectorPlacement.EquallySpacedRectSide\",\"uuid\":\"e6d1833a-8836-49de-81ae-600a650351e4\"},{\"content\":{\"connectorIds\":[\"Out1\"],\"side\":\"RIGHT\"},\"type\":\"ConnectorPlacement.EquallySpacedRectSide\",\"uuid\":\"f245f6bb-811b-4e93-b151-5c323e86052c\"},{\"content\":{\"side\":\"TOP\"},\"type\":\"ConnectorPlacement.EquallySpacedRectSide\",\"uuid\":\"48a167ed-d4c2-4e7f-a44b-e328bb65996f\"}]},\"type\":\"ConnectorPlacement.EquallySpacedConnector\",\"uuid\":\"b7272ec2-108a-4004-85a9-2681fa300cc3\"}],\"packageUris\":[\"http://schema.mathworks.com/mf0/Connector/R2020b\"],\"version\":\"1.0\"}"
  Bus Element Out1 : Outport  PortName=PipeDetectionResult
  Bus Element Out2 : Outport  Port=2  PortName=FaultDetectionResult
  wires:
  Bus Element In1/1 -> CamStarting/1(AUVPipeDistance)
  Bus Element In5/1 -> XrayStarting/1(AUVPipeDistance)
  CamStarting/1(BinarySignal) -> PipeDetection/1(BinarySignal)
  XrayStarting/1(BinarySignal) -> FaultDetection/1(BinarySignal)
  PipeDetection/1(PipeDetectionResult) -> Bus Element Out1/1
  FaultDetection/1(FaultDetectionResult) -> Bus Element Out2/1
  Bus Element In3/1 -> PipeDetection/2(PipeDetectionTrainedModel)
  Bus Element In4/1 -> FaultDetection/2(FaultDetectionTrainedModel)

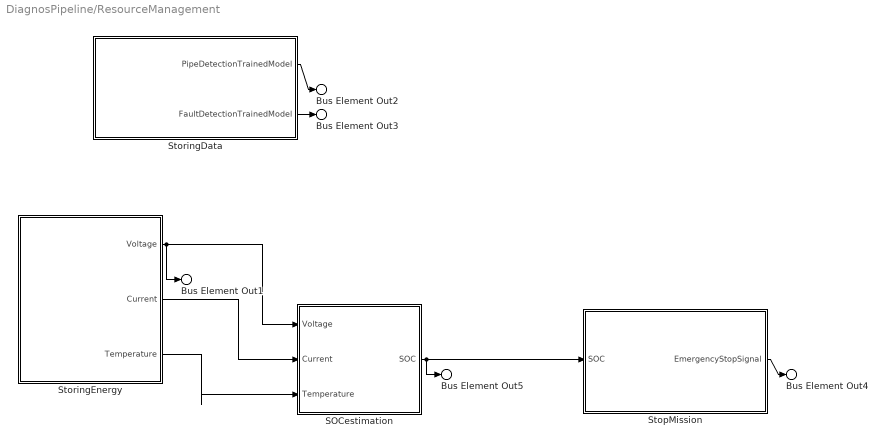
== system DiagnosPipeline/ResourceManagement ==
  SOCestimation : Subsystem
      settings: PortSchema="{\"entries\":[{\"content\":{\"headerSize\":26,\"margin\":15,\"minimumSpacing\":25,\"sides\":[{\"content\":{\"connectorIds\":[\"In1\",\"In2\",\"In3\"]},\"type\":\"ConnectorPlacement.EquallySpacedRectSide\",\"uuid\":\"e6d1833a-8836-49de-81ae-600a650351e4\"},{\"content\":{\"connectorIds\":[\"Out1\"],\"side\":\"RIGHT\"},\"type\":\"ConnectorPlacement.EquallySpacedRectSide\",\"uuid\":\"f245f6bb-811b-4e93-b151-5c323e86052c\"},{\"content\":{\"side\":\"TOP\"},\"type\":\"ConnectorPlacement.EquallySpacedRectSide\",\"uuid\":\"48a167ed-d4c2-4e7f-a44b-e328bb65996f\"}]},\"type\":\"ConnectorPlacement.EquallySpacedConnector\",\"uuid\":\"b7272ec2-108a-4004-85a9-2681fa300cc3\"}],\"packageUris\":[\"http://schema.mathworks.com/mf0/Connector/R2020b\"],\"version\":\"1.0\"}"
  StopMission : Subsystem
      settings: PortSchema="{\"entries\":[{\"content\":{\"headerSize\":26,\"margin\":15,\"minimumSpacing\":25,\"sides\":[{\"content\":{\"connectorIds\":[\"In1\"]},\"type\":\"ConnectorPlacement.EquallySpacedRectSide\",\"uuid\":\"f9fadc38-a5ed-4d2c-8740-325682f7523a\"},{\"content\":{\"connectorIds\":[\"Out1\"],\"side\":\"RIGHT\"},\"type\":\"ConnectorPlacement.EquallySpacedRectSide\",\"uuid\":\"4cbd6435-b8f9-40e4-9703-696d88d9d9ae\"},{\"content\":{\"side\":\"TOP\"},\"type\":\"ConnectorPlacement.EquallySpacedRectSide\",\"uuid\":\"4cdd59a8-5a6d-4988-b682-29bfa74ce39c\"}]},\"type\":\"ConnectorPlacement.EquallySpacedConnector\",\"uuid\":\"f6db6523-916a-4ed8-a308-4b7cb9d0bc19\"}],\"packageUris\":[\"http://schema.mathworks.com/mf0/Connector/R2020b\"],\"version\":\"1.0\"}"
  StoringData : Subsystem
      settings: PortSchema="{\"entries\":[{\"content\":{\"headerSize\":26,\"margin\":15,\"minimumSpacing\":25,\"sides\":[{\"content\":{},\"type\":\"ConnectorPlacement.EquallySpacedRectSide\",\"uuid\":\"e6d1833a-8836-49de-81ae-600a650351e4\"},{\"content\":{\"connectorIds\":[\"Out1\",\"Out2\"],\"side\":\"RIGHT\"},\"type\":\"ConnectorPlacement.EquallySpacedRectSide\",\"uuid\":\"f245f6bb-811b-4e93-b151-5c323e86052c\"},{\"content\":{\"side\":\"TOP\"},\"type\":\"ConnectorPlacement.EquallySpacedRectSide\",\"uuid\":\"48a167ed-d4c2-4e7f-a44b-e328bb65996f\"}]},\"type\":\"ConnectorPlacement.EquallySpacedConnector\",\"uuid\":\"b7272ec2-108a-4004-85a9-2681fa300cc3\"}],\"packageUris\":[\"http://schema.mathworks.com/mf0/Connector/R2020b\"],\"version\":\"1.0\"}"
  StoringEnergy : Subsystem
      settings: PortSchema="{\"entries\":[{\"content\":{\"headerSize\":26,\"margin\":15,\"minimumSpacing\":25,\"sides\":[{\"content\":{},\"type\":\"ConnectorPlacement.EquallySpacedRectSide\",\"uuid\":\"e6d1833a-8836-49de-81ae-600a650351e4\"},{\"content\":{\"connectorIds\":[\"Out1\",\"Out2\",\"Out3\"],\"side\":\"RIGHT\"},\"type\":\"ConnectorPlacement.EquallySpacedRectSide\",\"uuid\":\"f245f6bb-811b-4e93-b151-5c323e86052c\"},{\"content\":{\"side\":\"TOP\"},\"type\":\"ConnectorPlacement.EquallySpacedRectSide\",\"uuid\":\"48a167ed-d4c2-4e7f-a44b-e328bb65996f\"}]},\"type\":\"ConnectorPlacement.EquallySpacedConnector\",\"uuid\":\"b7272ec2-108a-4004-85a9-2681fa300cc3\"}],\"packageUris\":[\"http://schema.mathworks.com/mf0/Connector/R2020b\"],\"version\":\"1.0\"}"
  Bus Element Out2 : Outport  PortName=PipeDetectionTrainedModel
  Bus Element Out3 : Outport  Port=2  PortName=FaultDetectionTrainedModel
  Bus Element Out5 : Outport  Port=3  PortName=SOC
  Bus Element Out1 : Outport  Port=4  PortName=Voltage
  Bus Element Out4 : Outport  Port=5  PortName=EmergencyStopSignal
  wires:
  StoringData/1(PipeDetectionTrainedModel) -> Bus Element Out2/1
  StoringData/2(FaultDetectionTrainedModel) -> Bus Element Out3/1
  StopMission/1(EmergencyStopSignal) -> Bus Element Out4/1
  SOCestimation/1(SOC) -> Bus Element Out5/1, StopMission/1(SOC)
  StoringEnergy/1(Voltage) -> Bus Element Out1/1, SOCestimation/1(Voltage)
  StoringEnergy/2(Current) -> SOCestimation/2(Current)
  StoringEnergy/3(Temperature) -> SOCestimation/3(Temperature)

== system DiagnosPipeline/StakeReq ==
  Bus Element In1 : Inport  PortName=Oceanic Environment
  Bus Element In2 : Inport  Port=2  PortName=DisrepaireSignal
  EnvironmentProtection : Subsystem
      settings: PortSchema="{\"entries\":[{\"content\":{\"headerSize\":26,\"margin\":15,\"minimumSpacing\":25,\"sides\":[{\"content\":{\"connectorIds\":[\"In1\"]},\"type\":\"ConnectorPlacement.EquallySpacedRectSide\",\"uuid\":\"f9fadc38-a5ed-4d2c-8740-325682f7523a\"},{\"content\":{\"side\":\"RIGHT\"},\"type\":\"ConnectorPlacement.EquallySpacedRectSide\",\"uuid\":\"4cbd6435-b8f9-40e4-9703-696d88d9d9ae\"},{\"content\":{\"side\":\"TOP\"},\"type\":\"ConnectorPlacement.EquallySpacedRectSide\",\"uuid\":\"4cdd59a8-5a6d-4988-b682-29bfa74ce39c\"}]},\"type\":\"ConnectorPlacement.EquallySpacedConnector\",\"uuid\":\"f6db6523-916a-4ed8-a308-4b7cb9d0bc19\"}],\"packageUris\":[\"http://schema.mathworks.com/mf0/Connector/R2020b\"],\"version\":\"1.0\"}"
  Maintenance : Subsystem
      settings: PortSchema="{\"entries\":[{\"content\":{\"headerSize\":26,\"margin\":15,\"minimumSpacing\":25,\"sides\":[{\"content\":{\"connectorIds\":[\"In1\"]},\"type\":\"ConnectorPlacement.EquallySpacedRectSide\",\"uuid\":\"f9fadc38-a5ed-4d2c-8740-325682f7523a\"},{\"content\":{\"side\":\"RIGHT\"},\"type\":\"ConnectorPlacement.EquallySpacedRectSide\",\"uuid\":\"4cbd6435-b8f9-40e4-9703-696d88d9d9ae\"},{\"content\":{\"side\":\"TOP\"},\"type\":\"ConnectorPlacement.EquallySpacedRectSide\",\"uuid\":\"4cdd59a8-5a6d-4988-b682-29bfa74ce39c\"}]},\"type\":\"ConnectorPlacement.EquallySpacedConnector\",\"uuid\":\"f6db6523-916a-4ed8-a308-4b7cb9d0bc19\"}],\"packageUris\":[\"http://schema.mathworks.com/mf0/Connector/R2020b\"],\"version\":\"1.0\"}"
  wires:
  Bus Element In1/1 -> EnvironmentProtection/1(Oceanic Environment)
  Bus Element In2/1 -> Maintenance/1(DisrepaireSignal)

== system DiagnosPipeline/DataCommunication/Decryption ==
  Bus Element In1 : Inport  PortName=MissionSignal
  Bus Element Out1 : Outport  PortName=MissionMessage

== system DiagnosPipeline/DataCommunication/Encryption ==
  Bus Element In1 : Inport  PortName=LogSignal
  Bus Element Out1 : Outport  PortName=LogSignalEncrypted

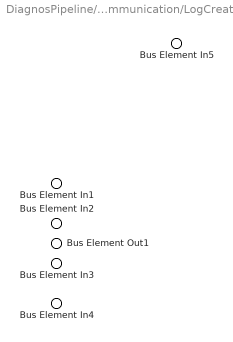
== system DiagnosPipeline/DataCommunication/LogCreation ==
  Bus Element In1 : Inport  PortName=PipeDetectionResult
  Bus Element In2 : Inport  Port=2  PortName=FaultDetectionResult
  Bus Element In5 : Inport  Port=3  PortName=SOC
  Bus Element In3 : Inport  Port=4  PortName=PoseConfiguration
  Bus Element In4 : Inport  Port=5  PortName=EmergencyStop
  Bus Element Out1 : Outport  PortName=LogSignal

== system DiagnosPipeline/DataCommunication/ReceivingData ==
  Bus Element In1 : Inport  PortName=Mission Signal
  Bus Element Out1 : Outport  PortName=MissionSignal

== system DiagnosPipeline/DataCommunication/SendingData ==
  Bus Element In1 : Inport  PortName=LogSignalEncrypted
  Bus Element Out1 : Outport  PortName=LogSignalEncryptedToLS

== system DiagnosPipeline/KeepSafety/PressureResistance ==
  Bus Element In1 : Inport  PortName=Oceanic Environment

== system DiagnosPipeline/KeepSafety/PulseGeneration ==
  Bus Element Out1 : Outport  PortName=Pulse

== system DiagnosPipeline/KeepSafety/SalinityResistance ==
  Bus Element In1 : Inport  PortName=Oceanic Environment

== system DiagnosPipeline/KeepSafety/WaterResistance ==
  Bus Element In1 : Inport  PortName=Oceanic Environment

== system DiagnosPipeline/Localization/IMUseperator ==
  Bus Element In1 : Inport  PortName=InertialMeasurement
  Bus Element Out1 : Outport  PortName=Pressure
  Bus Element Out2 : Outport  Port=2  PortName=Omega
  Bus Element Out3 : Outport  Port=3  PortName=Acceleration

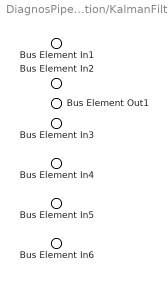
== system DiagnosPipeline/Localization/KalmanFilter ==
  Bus Element In1 : Inport  PortName=Lat
  Bus Element In2 : Inport  Port=2  PortName=Long
  Bus Element In3 : Inport  Port=3  PortName=Alt
  Bus Element In4 : Inport  Port=4  PortName=Pressure
  Bus Element In5 : Inport  Port=5  PortName=Omega
  Bus Element In6 : Inport  Port=6  PortName=Acceleration
  Bus Element Out1 : Outport  PortName=PoseConfiguration

== system DiagnosPipeline/Localization/MeasureInertial ==
  Bus Element In2 : Inport  PortName=Gravity
  Bus Element Out1 : Outport  PortName=InertialMeasurement

== system DiagnosPipeline/Localization/MeasurePose ==
  Bus Element In1 : Inport  PortName=Satellite
  Bus Element Out1 : Outport  PortName=NMEA

== system DiagnosPipeline/Localization/Seperator ==
  Bus Element In1 : Inport  PortName=NMEA
  Bus Element Out1 : Outport  PortName=Lat
  Bus Element Out2 : Outport  Port=2  PortName=Long
  Bus Element Out3 : Outport  Port=3  PortName=Alt

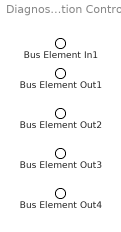
== system DiagnosPipeline/MotionControl/Motion Control ==
  Bus Element In1 : Inport  PortName=TrajectoryMessage
  Bus Element Out1 : Outport  PortName=ControlSignal1
  Bus Element Out2 : Outport  Port=2  PortName=ControlSignal2
  Bus Element Out3 : Outport  Port=3  PortName=ControlSignal3
  Bus Element Out4 : Outport  Port=4  PortName=ControlSignal4

== system DiagnosPipeline/MotionControl/RotateMotor1 ==
  Bus Element In2 : Inport  PortName=Energy
  Bus Element In1 : Inport  Port=2  PortName=ControlSignal1

== system DiagnosPipeline/MotionControl/RotateMotor2 ==
  Bus Element In2 : Inport  PortName=Energy
  Bus Element In1 : Inport  Port=2  PortName=ControlSignal2

== system DiagnosPipeline/MotionControl/RotateMotor3 ==
  Bus Element In2 : Inport  PortName=Energy
  Bus Element In1 : Inport  Port=2  PortName=ControlSignal3

== system DiagnosPipeline/MotionControl/RotateMotor4 ==
  Bus Element In2 : Inport  PortName=Energy
  Bus Element In1 : Inport  Port=2  PortName=ControlSignal4

== system DiagnosPipeline/PipelineDiagnosis/CamStarting ==
  Bus Element In1 : Inport  PortName=AUVPipeDistance
  Bus Element Out1 : Outport  PortName=BinarySignal

== system DiagnosPipeline/PipelineDiagnosis/FaultDetection ==
  Bus Element In1 : Inport  PortName=BinarySignal
  Bus Element In2 : Inport  Port=2  PortName=FaultDetectionTrainedModel
  Bus Element Out1 : Outport  PortName=FaultDetectionResult

== system DiagnosPipeline/PipelineDiagnosis/PipeDetection ==
  Bus Element In1 : Inport  PortName=BinarySignal
  Bus Element In2 : Inport  Port=2  PortName=PipeDetectionTrainedModel
  Bus Element Out2 : Outport  PortName=PipeDetectionResult

== system DiagnosPipeline/PipelineDiagnosis/XrayStarting ==
  Bus Element In1 : Inport  PortName=AUVPipeDistance
  Bus Element Out1 : Outport  PortName=BinarySignal

== system DiagnosPipeline/ResourceManagement/SOCestimation ==
  Bus Element In1 : Inport  PortName=Voltage
  Bus Element In2 : Inport  Port=2  PortName=Current
  Bus Element In3 : Inport  Port=3  PortName=Temperature
  Bus Element Out1 : Outport  PortName=SOC

== system DiagnosPipeline/ResourceManagement/StopMission ==
  Bus Element In1 : Inport  PortName=SOC
  Bus Element Out1 : Outport  PortName=EmergencyStopSignal

== system DiagnosPipeline/ResourceManagement/StoringData ==
  Bus Element Out1 : Outport  PortName=PipeDetectionTrainedModel
  Bus Element Out2 : Outport  Port=2  PortName=FaultDetectionTrainedModel

== system DiagnosPipeline/ResourceManagement/StoringEnergy ==
  Bus Element Out1 : Outport  PortName=Voltage
  Bus Element Out2 : Outport  Port=2  PortName=Current
  Bus Element Out3 : Outport  Port=3  PortName=Temperature

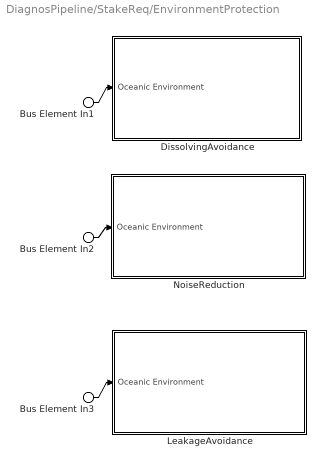
== system DiagnosPipeline/StakeReq/EnvironmentProtection ==
  Bus Element In1 : Inport  PortName=Oceanic Environment
  Bus Element In2 : Inport  PortName=Oceanic Environment
  Bus Element In3 : Inport  PortName=Oceanic Environment
  DissolvingAvoidance : Subsystem
      settings: PortSchema="{\"entries\":[{\"content\":{\"headerSize\":26,\"margin\":15,\"minimumSpacing\":25,\"sides\":[{\"content\":{\"connectorIds\":[\"In1\"]},\"type\":\"ConnectorPlacement.EquallySpacedRectSide\",\"uuid\":\"f9fadc38-a5ed-4d2c-8740-325682f7523a\"},{\"content\":{\"side\":\"RIGHT\"},\"type\":\"ConnectorPlacement.EquallySpacedRectSide\",\"uuid\":\"4cbd6435-b8f9-40e4-9703-696d88d9d9ae\"},{\"content\":{\"side\":\"TOP\"},\"type\":\"ConnectorPlacement.EquallySpacedRectSide\",\"uuid\":\"4cdd59a8-5a6d-4988-b682-29bfa74ce39c\"}]},\"type\":\"ConnectorPlacement.EquallySpacedConnector\",\"uuid\":\"f6db6523-916a-4ed8-a308-4b7cb9d0bc19\"}],\"packageUris\":[\"http://schema.mathworks.com/mf0/Connector/R2020b\"],\"version\":\"1.0\"}"
  LeakageAvoidance : Subsystem
      settings: PortSchema="{\"entries\":[{\"content\":{\"headerSize\":26,\"margin\":15,\"minimumSpacing\":25,\"sides\":[{\"content\":{\"connectorIds\":[\"In1\"]},\"type\":\"ConnectorPlacement.EquallySpacedRectSide\",\"uuid\":\"f9fadc38-a5ed-4d2c-8740-325682f7523a\"},{\"content\":{\"side\":\"RIGHT\"},\"type\":\"ConnectorPlacement.EquallySpacedRectSide\",\"uuid\":\"4cbd6435-b8f9-40e4-9703-696d88d9d9ae\"},{\"content\":{\"side\":\"TOP\"},\"type\":\"ConnectorPlacement.EquallySpacedRectSide\",\"uuid\":\"4cdd59a8-5a6d-4988-b682-29bfa74ce39c\"}]},\"type\":\"ConnectorPlacement.EquallySpacedConnector\",\"uuid\":\"f6db6523-916a-4ed8-a308-4b7cb9d0bc19\"}],\"packageUris\":[\"http://schema.mathworks.com/mf0/Connector/R2020b\"],\"version\":\"1.0\"}"
  NoiseReduction : Subsystem
      settings: PortSchema="{\"entries\":[{\"content\":{\"headerSize\":26,\"margin\":15,\"minimumSpacing\":25,\"sides\":[{\"content\":{\"connectorIds\":[\"In1\"]},\"type\":\"ConnectorPlacement.EquallySpacedRectSide\",\"uuid\":\"f9fadc38-a5ed-4d2c-8740-325682f7523a\"},{\"content\":{\"side\":\"RIGHT\"},\"type\":\"ConnectorPlacement.EquallySpacedRectSide\",\"uuid\":\"4cbd6435-b8f9-40e4-9703-696d88d9d9ae\"},{\"content\":{\"side\":\"TOP\"},\"type\":\"ConnectorPlacement.EquallySpacedRectSide\",\"uuid\":\"4cdd59a8-5a6d-4988-b682-29bfa74ce39c\"}]},\"type\":\"ConnectorPlacement.EquallySpacedConnector\",\"uuid\":\"f6db6523-916a-4ed8-a308-4b7cb9d0bc19\"}],\"packageUris\":[\"http://schema.mathworks.com/mf0/Connector/R2020b\"],\"version\":\"1.0\"}"
  wires:
  Bus Element In1/1 -> DissolvingAvoidance/1(Oceanic Environment)
  Bus Element In2/1 -> NoiseReduction/1(Oceanic Environment)
  Bus Element In3/1 -> LeakageAvoidance/1(Oceanic Environment)

== system DiagnosPipeline/StakeReq/Maintenance ==
  Bus Element In1 : Inport  PortName=DisrepaireSignal
  Bus Element In2 : Inport  PortName=DisrepaireSignal
  Disassembly : Subsystem
      settings: PortSchema="{\"entries\":[{\"content\":{\"headerSize\":26,\"margin\":15,\"minimumSpacing\":25,\"sides\":[{\"content\":{\"connectorIds\":[\"In1\"]},\"type\":\"ConnectorPlacement.EquallySpacedRectSide\",\"uuid\":\"f9fadc38-a5ed-4d2c-8740-325682f7523a\"},{\"content\":{\"side\":\"RIGHT\"},\"type\":\"ConnectorPlacement.EquallySpacedRectSide\",\"uuid\":\"4cbd6435-b8f9-40e4-9703-696d88d9d9ae\"},{\"content\":{\"side\":\"TOP\"},\"type\":\"ConnectorPlacement.EquallySpacedRectSide\",\"uuid\":\"4cdd59a8-5a6d-4988-b682-29bfa74ce39c\"}]},\"type\":\"ConnectorPlacement.EquallySpacedConnector\",\"uuid\":\"f6db6523-916a-4ed8-a308-4b7cb9d0bc19\"}],\"packageUris\":[\"http://schema.mathworks.com/mf0/Connector/R2020b\"],\"version\":\"1.0\"}"
  Replacement : Subsystem
      settings: PortSchema="{\"entries\":[{\"content\":{\"headerSize\":26,\"margin\":15,\"minimumSpacing\":25,\"sides\":[{\"content\":{\"connectorIds\":[\"In1\"]},\"type\":\"ConnectorPlacement.EquallySpacedRectSide\",\"uuid\":\"f9fadc38-a5ed-4d2c-8740-325682f7523a\"},{\"content\":{\"side\":\"RIGHT\"},\"type\":\"ConnectorPlacement.EquallySpacedRectSide\",\"uuid\":\"4cbd6435-b8f9-40e4-9703-696d88d9d9ae\"},{\"content\":{\"side\":\"TOP\"},\"type\":\"ConnectorPlacement.EquallySpacedRectSide\",\"uuid\":\"4cdd59a8-5a6d-4988-b682-29bfa74ce39c\"}]},\"type\":\"ConnectorPlacement.EquallySpacedConnector\",\"uuid\":\"f6db6523-916a-4ed8-a308-4b7cb9d0bc19\"}],\"packageUris\":[\"http://schema.mathworks.com/mf0/Connector/R2020b\"],\"version\":\"1.0\"}"
  wires:
  Bus Element In1/1 -> Disassembly/1(DisrepaireSignal)
  Bus Element In2/1 -> Replacement/1(DisrepaireSignal)

== system DiagnosPipeline/StakeReq/EnvironmentProtection/DissolvingAvoidance ==
  Bus Element In1 : Inport  PortName=Oceanic Environment

== system DiagnosPipeline/StakeReq/EnvironmentProtection/LeakageAvoidance ==
  Bus Element In1 : Inport  PortName=Oceanic Environment

== system DiagnosPipeline/StakeReq/EnvironmentProtection/NoiseReduction ==
  Bus Element In1 : Inport  PortName=Oceanic Environment

== system DiagnosPipeline/StakeReq/Maintenance/Disassembly ==
  Bus Element In1 : Inport  PortName=DisrepaireSignal

== system DiagnosPipeline/StakeReq/Maintenance/Replacement ==
  Bus Element In1 : Inport  PortName=DisrepaireSignal
